simulink model "Quest"  (R2024b)
settings: Solver=VariableStepAuto  StartTime=0.0  StopTime=10.0  RelTol=1e-3
undefined symbols (not defined in the file or in its folder): magnitude
libraries: aerolibutil x1
settings Model: Creator=prani  LastModifiedBy=prani

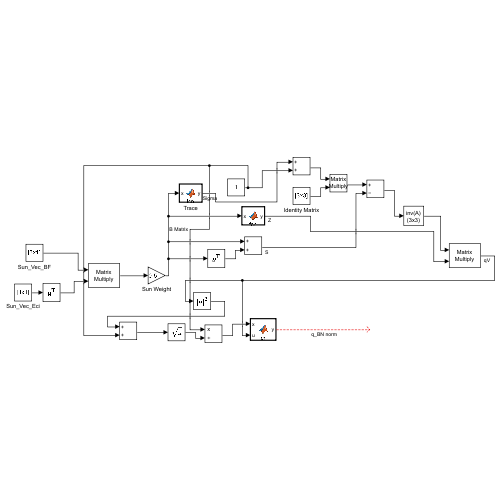
[thumbnail: Simulink's stored preview of the top-level diagram]
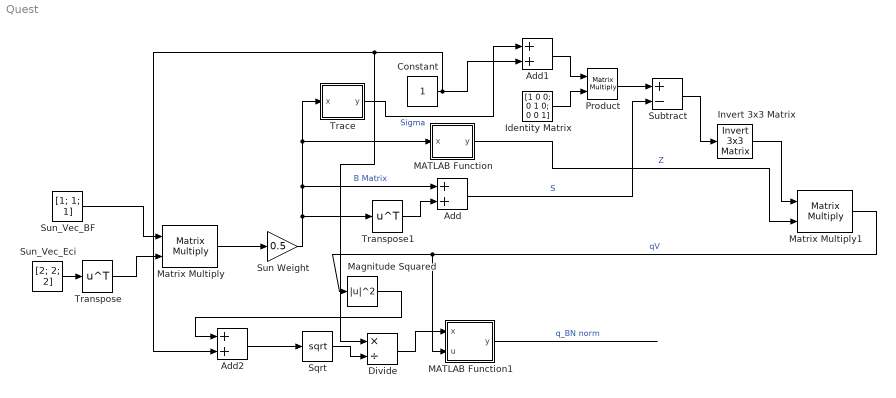
== system Quest ==
  Add : Sum
  Add1 : Sum
  Add2 : Sum
  Constant : Constant
  Divide : Product  Inputs=*/
  Identity Matrix : Constant  Value=[1 0 0; 0 1 0; 0 0 1]
  Invert 3x3 Matrix : aerolibutil/Invert  3x3 Matrix
  MATLAB Function : MATLAB Function  TreatAsAtomicUnit=on
  MATLAB Function1 : MATLAB Function  TreatAsAtomicUnit=on
  Magnitude Squared : Math  Operator=magnitude^2
  Matrix Multiply : Product  Multiplication=Matrix(*)
  Matrix Multiply1 : Product  Multiplication=Matrix(*)
  Product : Product  Multiplication=Matrix(*)
  Sqrt : Sqrt
  Subtract : Sum  Inputs=+-
  Sun Weight : Gain  Gain=0.5
  Sun_Vec_BF : Constant  Value=[1; 1; 1]
  Sun_Vec_Eci : Constant  Value=[2; 2; 2]
  Trace : MATLAB Function  TreatAsAtomicUnit=on
  Transpose : Math  Operator=transpose
  Transpose1 : Math  Operator=transpose
  wires:
  Sun_Vec_Eci/1 -> Transpose/1
  Transpose/1 -> Matrix Multiply/2
  Sun_Vec_BF/1 -> Matrix Multiply/1
  Matrix Multiply/1 -> Sun Weight/1
  Sun Weight/1 -> Transpose1/1, Add/1, Trace/1(x), MATLAB Function/1(x)  "B Matrix"
  Transpose1/1 -> Add/2
  Trace/1(y) -> Add1/1  "Sigma"
  Add/1 -> Subtract/2  "S"
  MATLAB Function/1(y) -> Matrix Multiply1/2  "Z"
  Identity Matrix/1 -> Product/2
  Add1/1 -> Product/1
  Product/1 -> Subtract/1
  Subtract/1 -> Invert 3x3 Matrix/1
  Invert 3x3 Matrix/1 -> Matrix Multiply1/1
  Constant/1 -> Divide/1, Add2/2, Add1/2
  Add2/1 -> Sqrt/1
  Matrix Multiply1/1 -> MATLAB Function1/2(u), Magnitude Squared/1  "qV"
  Magnitude Squared/1 -> Add2/1
  Sqrt/1 -> Divide/2
  Divide/1 -> MATLAB Function1/1(x)
  MATLAB Function1/1(y) -> ?  "q_BN norm"

== matlab function Quest/Trace ==
  data: x input; y output
function y = fcn(x)

y=x(1,1)+x(2,2)+x(3,3);

== matlab function Quest/MATLAB Function1 ==
  data: x input; u input; y output
function y = fcn(x,u)

%x is a scalar, u is the 3x1 vector

y=x*[1;u];

== matlab function Quest/MATLAB Function ==
  data: x input; y output
function y = fcn(x)

y(1)=x(2,3)-x(3,2);
y(2)=x(3,1)-x(1,3);
y(3)=x(1,2)-x(2,1);
